simulink model "SfastModelFFA"  (R2023a)
settings: Solver=VariableStepAuto  StartTime=0.0  StopTime=150  RelTol=1e-3
libraries: cstblocks x12
settings Model: Creator=jprmj  LastModifiedBy=juan
settings OptimizationCC: ReuseModelBlockBuffer=off

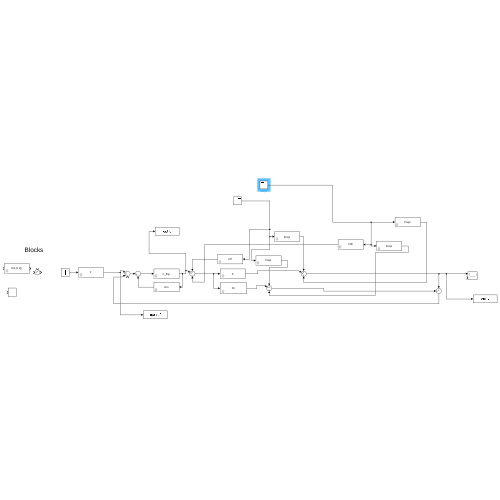
[thumbnail: Simulink's stored preview of the top-level diagram]
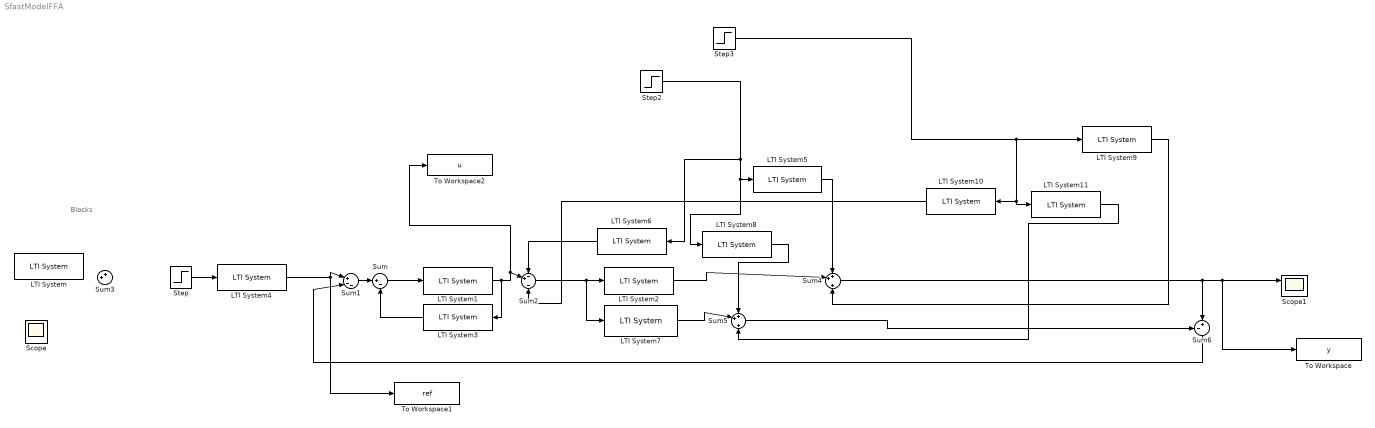
== system SfastModelFFA ==
  note: Blocks
  LTI System : cstblocks/LTI System  sys=tf(1,[1 1])  IC=[]
  LTI System1 : cstblocks/LTI System  sys=C_ffsp  IC=[]
  LTI System10 : cstblocks/LTI System  sys=Cff2  IC=[]
  LTI System11 : cstblocks/LTI System  sys=Pnq2  IC=[]
  LTI System2 : cstblocks/LTI System  sys=P  IC=[]
  LTI System3 : cstblocks/LTI System  sys=Gm  IC=[]
  LTI System4 : cstblocks/LTI System  sys=F  IC=[]
  LTI System5 : cstblocks/LTI System  sys=Pnq1  IC=[]
  LTI System6 : cstblocks/LTI System  sys=Cff  IC=[]
  LTI System7 : cstblocks/LTI System  sys=Pn  IC=[]
  LTI System8 : cstblocks/LTI System  sys=Pnq1  IC=[]
  LTI System9 : cstblocks/LTI System  sys=Pnq2  IC=[]
  Scope : Scope
  Scope1 : Scope  NumInputPorts=2
  Step : Step  SampleTime=0
  Step2 : Step  After=500  SampleTime=50
  Step3 : Step  After=-4  SampleTime=100
  Sum : Sum  Inputs=|+-
  Sum1 : Sum  Inputs=|+--
  Sum2 : Sum  Inputs=-+|-
  Sum3 : Sum  Inputs=++|
  Sum4 : Sum  Inputs=++|+
  Sum5 : Sum  Inputs=++|+
  Sum6 : Sum  Inputs=-+|
  To Workspace : ToWorkspace  VariableName=y  SaveFormat=Timeseries  SampleTime=-1
  To Workspace1 : ToWorkspace  VariableName=ref  SaveFormat=Timeseries  SampleTime=-1
  To Workspace2 : ToWorkspace  VariableName=u  SaveFormat=Timeseries  SampleTime=-1
  wires:
  Sum2/1 -> LTI System7/1, LTI System2/1
  LTI System1/1 -> LTI System3/1, To Workspace2/1, Sum2/2
  LTI System3/1 -> Sum/2
  LTI System4/1 -> To Workspace1/1, Sum1/1
  LTI System2/1 -> Sum4/2
  LTI System5/1 -> Sum4/1
  LTI System6/1 -> Sum2/1
  LTI System7/1 -> Sum5/2
  LTI System8/1 -> Sum5/1
  LTI System11/1 -> Sum5/3
  Sum5/1 -> Sum6/1
  Sum4/1 -> Sum6/2, To Workspace/1, Scope1/1
  Step3/1 -> LTI System10/1, LTI System11/1, LTI System9/1
  Step2/1 -> LTI System6/1, LTI System8/1, LTI System5/1
  LTI System9/1 -> Sum4/3
  LTI System10/1 -> Sum2/3
  Sum1/1 -> Sum/1
  Sum6/1 -> Sum1/2
  Sum/1 -> LTI System1/1
  Step/1 -> LTI System4/1
